simulink library "halout"  (R2021b)
settings: Solver=VariableStepAuto  StartTime=0.0  StopTime=10.0  RelTol=1e-3
undefined symbols (not defined in the file): C_TASK_5MS_S, FALSE, KHAL_CAN1FDAPS3E2E_flg, KHAL_CAN1FDAPS3TxReq_flg, KHAL_CAN1FDVCU2E2E_flg, KHAL_CAN1FDVCU2TxReq_flg, KHAL_CAN1FDVCU3E2E_flg, KHAL_CAN1FDVCU3TxReq_flg, KHAL_CAN1TxReq_flg, KHAL_CAN2TxReq_flg, KHAL_CAN3FDVCU1TxReq_flg, KHAL_CAN3FDVCU2E2E_flg, KHAL_CAN3FDVCU2TxReq_flg, KHAL_CAN3TxReq_flg, KHAL_CAN4FDVCU1E2E_flg, KHAL_CAN4FDVCU1TxReq_flg, KHAL_CAN4TxReq_flg, KHAL_CAN5TxReq_flg, ONE_INT, TRUE, ZERO_INT
libraries: FVT_lib x383, simulink x179
(part 20 of 20)

== system halout/HAL_OUT/CAN5/FD_VCU0_0x1F0/PwrStaSelect ==
  PwrStaSelect : Inport
  Data Type Conversion : DataTypeConversion  OutDataTypeStr=uint8  RndMeth=Round
  CAN5_PwrStaSelect : Outport
  wires:
  Data Type Conversion/1 -> CAN5_PwrStaSelect/1
  PwrStaSelect/1 -> Data Type Conversion/1

== system halout/HAL_OUT/CAN5/FD_VCU0_0x1F0/PwrStaTOSta ==
  PwrStaTOSta : Inport
  Data Type Conversion : DataTypeConversion  OutDataTypeStr=uint8  RndMeth=Round
  CAN5_PwrStaTOSta : Outport
  wires:
  Data Type Conversion/1 -> CAN5_PwrStaTOSta/1
  PwrStaTOSta/1 -> Data Type Conversion/1

== system halout/HAL_OUT/CAN5/FD_VCU0_0x1F0/PwrUpReq ==
  PwrUpReq : Inport
  Data Type Conversion : DataTypeConversion  OutDataTypeStr=uint8  RndMeth=Round
  CAN5_PwrUpReq : Outport
  wires:
  Data Type Conversion/1 -> CAN5_PwrUpReq/1
  PwrUpReq/1 -> Data Type Conversion/1

== system halout/HAL_OUT/CAN5/FD_VCU0_0x1F0/RrTqSource ==
  RrTqSource : Inport
  Data Type Conversion : DataTypeConversion  OutDataTypeStr=uint8  RndMeth=Round
  CAN5_Rr_TqSource : Outport
  wires:
  Data Type Conversion/1 -> CAN5_Rr_TqSource/1
  RrTqSource/1 -> Data Type Conversion/1

== system halout/HAL_OUT/CAN5/FD_VCU0_0x1F0/SchedChgTOSta ==
  SchedChgTOSta : Inport
  Data Type Conversion : DataTypeConversion  OutDataTypeStr=uint8  RndMeth=Round
  CAN5_SchedChgTOSta : Outport
  wires:
  Data Type Conversion/1 -> CAN5_SchedChgTOSta/1
  SchedChgTOSta/1 -> Data Type Conversion/1

== system halout/HAL_OUT/CAN5/FD_VCU0_0x1F0/SilentChkAllowSleep ==
  SilentChkAllowSleep : Inport
  Data Type Conversion : DataTypeConversion  OutDataTypeStr=uint8  RndMeth=Round
  CAN5_SilentChkAllowSleep : Outport
  wires:
  Data Type Conversion/1 -> CAN5_SilentChkAllowSleep/1
  SilentChkAllowSleep/1 -> Data Type Conversion/1

== system halout/HAL_OUT/CAN5/FD_VCU0_0x1F0/SysAllowReadySta ==
  SysAllowReadySta : Inport
  Data Type Conversion : DataTypeConversion  OutDataTypeStr=uint8  RndMeth=Round
  CAN5_SysAllowReadySta : Outport
  wires:
  Data Type Conversion/1 -> CAN5_SysAllowReadySta/1
  SysAllowReadySta/1 -> Data Type Conversion/1

== system halout/HAL_OUT/CAN5/FD_VCU0_0x1F0/SysPwrSta ==
  SysPwrSta : Inport
  Data Type Conversion : DataTypeConversion  OutDataTypeStr=uint8  RndMeth=Round
  CAN5_SysPwrSta : Outport
  wires:
  Data Type Conversion/1 -> CAN5_SysPwrSta/1
  SysPwrSta/1 -> Data Type Conversion/1

== system halout/HAL_OUT/CAN5/FD_VCU0_0x1F0/TCountSta ==
  TCountSta : Inport
  Data Type Conversion : DataTypeConversion  OutDataTypeStr=uint8  RndMeth=Round
  CAN5_TCountSta : Outport
  wires:
  Data Type Conversion/1 -> CAN5_TCountSta/1
  TCountSta/1 -> Data Type Conversion/1

== system halout/HAL_OUT/CAN5/FD_VCU0_0x1F0/TimerAllowSleep ==
  TimerAllowSleep : Inport
  Data Type Conversion : DataTypeConversion  OutDataTypeStr=uint8  RndMeth=Round
  CAN5_TimerAllowSleep : Outport
  wires:
  Data Type Conversion/1 -> CAN5_TimerAllowSleep/1
  TimerAllowSleep/1 -> Data Type Conversion/1

== system halout/HAL_OUT/CAN5/FD_VCU0_0x1F0/VCUBrkSWSta ==
  VCUBrkSWSta : Inport
  Data Type Conversion : DataTypeConversion  OutDataTypeStr=uint8  RndMeth=Round
  CAN5_VCUBrkSWSta : Outport
  wires:
  Data Type Conversion/1 -> CAN5_VCUBrkSWSta/1
  VCUBrkSWSta/1 -> Data Type Conversion/1

== system halout/HAL_OUT/CAN5/FD_VCU0_0x1F0/VCUFLDoorSta ==
  VCUFLDoorSta : Inport
  Data Type Conversion : DataTypeConversion  OutDataTypeStr=uint8  RndMeth=Round
  CAN5_VCUFLDoorSta : Outport
  wires:
  Data Type Conversion/1 -> CAN5_VCUFLDoorSta/1
  VCUFLDoorSta/1 -> Data Type Conversion/1

== system halout/HAL_OUT/CAN5/FD_VCU0_0x1F0/VCUFRDoorSta ==
  VCUFRDoorSta : Inport
  Data Type Conversion : DataTypeConversion  OutDataTypeStr=uint8  RndMeth=Round
  CAN5_VCUFRDoorSta : Outport
  wires:
  Data Type Conversion/1 -> CAN5_VCUFRDoorSta/1
  VCUFRDoorSta/1 -> Data Type Conversion/1

== system halout/HAL_OUT/CAN5/FD_VCU0_0x1F0/VCURLDoorSta ==
  VCURLDoorSta : Inport
  Data Type Conversion : DataTypeConversion  OutDataTypeStr=uint8  RndMeth=Round
  CAN5_VCURLDoorSta : Outport
  wires:
  Data Type Conversion/1 -> CAN5_VCURLDoorSta/1
  VCURLDoorSta/1 -> Data Type Conversion/1

== system halout/HAL_OUT/CAN5/FD_VCU0_0x1F0/VCURRDoorSta ==
  VCURRDoorSta : Inport
  Data Type Conversion : DataTypeConversion  OutDataTypeStr=uint8  RndMeth=Round
  CAN5_VCURRDoorSta : Outport
  wires:
  Data Type Conversion/1 -> CAN5_VCURRDoorSta/1
  VCURRDoorSta/1 -> Data Type Conversion/1

== system halout/HAL_OUT/CAN5/FD_VCU0_0x1F0/VehHVPwrAvail4THCM ==
  VehHVPwrAvail4THCM : Inport
  Data Type Conversion : DataTypeConversion  OutDataTypeStr=uint8  RndMeth=Round
  convert_out : FVT_lib/hal/convert_out  gain=50  offset=0
  CAN5_VehHVPwrAvail4THCM : Outport
  wires:
  Data Type Conversion/1 -> CAN5_VehHVPwrAvail4THCM/1
  convert_out/1 -> Data Type Conversion/1
  VehHVPwrAvail4THCM/1 -> convert_out/1

== system halout/HAL_OUT/CAN5/FD_VCU1_0x116/MSACrlSta ==
  MSACrlSta : Inport
  Data Type Conversion : DataTypeConversion  OutDataTypeStr=uint8  RndMeth=Round
  CAN5_MSA_Crl_Sta : Outport
  wires:
  Data Type Conversion/1 -> CAN5_MSA_Crl_Sta/1
  MSACrlSta/1 -> Data Type Conversion/1

== system halout/HAL_OUT/CAN5/FD_VCU1_0x116/PwrSta ==
  PwrSta : Inport
  Data Type Conversion : DataTypeConversion  OutDataTypeStr=uint8  RndMeth=Round
  CAN5_PwrSta : Outport
  wires:
  Data Type Conversion/1 -> CAN5_PwrSta/1
  PwrSta/1 -> Data Type Conversion/1

== system halout/HAL_OUT/CAN5/FD_VCU1_0x116/ShiftGearPosn ==
  ShiftGearPosn : Inport
  Data Type Conversion : DataTypeConversion  OutDataTypeStr=uint8  RndMeth=Round
  CAN5_ShiftGearPosn : Outport
  wires:
  Data Type Conversion/1 -> CAN5_ShiftGearPosn/1
  ShiftGearPosn/1 -> Data Type Conversion/1

== system halout/HAL_OUT/CAN5/FD_VCU3_0x159/CSVCU3CAN1 ==
  CSVCU3CAN1 : Inport
  Data Type Conversion : DataTypeConversion  OutDataTypeStr=uint8  RndMeth=Round
  CAN5_CS_VCU3_CAN1 : Outport
  wires:
  Data Type Conversion/1 -> CAN5_CS_VCU3_CAN1/1
  CSVCU3CAN1/1 -> Data Type Conversion/1

== system halout/HAL_OUT/CAN5/FD_VCU3_0x159/EquivAccPedalSWSta ==
  EquivAccPedalSWSta : Inport
  Data Type Conversion : DataTypeConversion  OutDataTypeStr=uint8  RndMeth=Round
  CAN5_EquivAccPedalSWSta : Outport
  wires:
  Data Type Conversion/1 -> CAN5_EquivAccPedalSWSta/1
  EquivAccPedalSWSta/1 -> Data Type Conversion/1

== system halout/HAL_OUT/CAN5/FD_VCU3_0x159/FrEDUActTqValid ==
  FrEDUActTqValid : Inport
  Data Type Conversion : DataTypeConversion  OutDataTypeStr=uint8  RndMeth=Round
  CAN5_Fr_EDUActTqValid : Outport
  wires:
  Data Type Conversion/1 -> CAN5_Fr_EDUActTqValid/1
  FrEDUActTqValid/1 -> Data Type Conversion/1

== system halout/HAL_OUT/CAN5/FD_VCU3_0x159/FrEDUAvailBrkRgnTq ==
  FrEDUAvailBrkRgnTq : Inport
  Data Type Conversion : DataTypeConversion  OutDataTypeStr=uint16  RndMeth=Round
  convert_out : FVT_lib/hal/convert_out  gain=0.5  offset=-5300
  CAN5_Fr_EDUAvailBrkRgnTq : Outport
  wires:
  Data Type Conversion/1 -> CAN5_Fr_EDUAvailBrkRgnTq/1
  convert_out/1 -> Data Type Conversion/1
  FrEDUAvailBrkRgnTq/1 -> convert_out/1

== system halout/HAL_OUT/CAN5/FD_VCU3_0x159/FrEDUAvailBrkRgnTqValid ==
  FrEDUAvailBrkRgnTqValid : Inport
  Data Type Conversion : DataTypeConversion  OutDataTypeStr=uint8  RndMeth=Round
  CAN5_Fr_EDUAvailBrkRgnTqValid : Outport
  wires:
  Data Type Conversion/1 -> CAN5_Fr_EDUAvailBrkRgnTqValid/1
  FrEDUAvailBrkRgnTqValid/1 -> Data Type Conversion/1

== system halout/HAL_OUT/CAN5/FD_VCU3_0x159/FrEDURealARgnTq ==
  FrEDURealARgnTq : Inport
  Data Type Conversion : DataTypeConversion  OutDataTypeStr=uint16  RndMeth=Round
  convert_out : FVT_lib/hal/convert_out  gain=1  offset=-5300
  CAN5_Fr_EDURealARgnTq : Outport
  wires:
  Data Type Conversion/1 -> CAN5_Fr_EDURealARgnTq/1
  convert_out/1 -> Data Type Conversion/1
  FrEDURealARgnTq/1 -> convert_out/1

== system halout/HAL_OUT/CAN5/FD_VCU3_0x159/FrEDURealDrvOrBRgnTq ==
  FrEDURealDrvOrBRgnTq : Inport
  Data Type Conversion : DataTypeConversion  OutDataTypeStr=uint16  RndMeth=Round
  convert_out : FVT_lib/hal/convert_out  gain=0.5  offset=-5300
  CAN5_Fr_EDURealDrvOrBRgnTq : Outport
  wires:
  Data Type Conversion/1 -> CAN5_Fr_EDURealDrvOrBRgnTq/1
  convert_out/1 -> Data Type Conversion/1
  FrEDURealDrvOrBRgnTq/1 -> convert_out/1

== system halout/HAL_OUT/CAN5/FD_VCU3_0x159/FrEDURolRgnTqValid ==
  FrEDURolRgnTqValid : Inport
  Data Type Conversion : DataTypeConversion  OutDataTypeStr=uint8  RndMeth=Round
  CAN5_Fr_EDURolRgnTqValid : Outport
  wires:
  Data Type Conversion/1 -> CAN5_Fr_EDURolRgnTqValid/1
  FrEDURolRgnTqValid/1 -> Data Type Conversion/1

== system halout/HAL_OUT/CAN5/FD_VCU3_0x159/FrEDUSpd ==
  FrEDUSpd : Inport
  Data Type Conversion : DataTypeConversion  OutDataTypeStr=uint16  RndMeth=Round
  convert_out : FVT_lib/hal/convert_out  gain=1  offset=-2000
  CAN5_Fr_EDUSpd : Outport
  wires:
  Data Type Conversion/1 -> CAN5_Fr_EDUSpd/1
  convert_out/1 -> Data Type Conversion/1
  FrEDUSpd/1 -> convert_out/1

== system halout/HAL_OUT/CAN5/FD_VCU3_0x159/FrEDUSpdValid ==
  FrEDUSpdValid : Inport
  Data Type Conversion : DataTypeConversion  OutDataTypeStr=uint8  RndMeth=Round
  CAN5_Fr_EDUSpdValid : Outport
  wires:
  Data Type Conversion/1 -> CAN5_Fr_EDUSpdValid/1
  FrEDUSpdValid/1 -> Data Type Conversion/1

== system halout/HAL_OUT/CAN5/FD_VCU3_0x159/FrRgnDecrSta ==
  FrRgnDecrSta : Inport
  Data Type Conversion : DataTypeConversion  OutDataTypeStr=uint8  RndMeth=Round
  CAN5_Fr_RgnDecrSta : Outport
  wires:
  Data Type Conversion/1 -> CAN5_Fr_RgnDecrSta/1
  FrRgnDecrSta/1 -> Data Type Conversion/1

== system halout/HAL_OUT/CAN5/FD_VCU3_0x159/FrRgnPermSta ==
  FrRgnPermSta : Inport
  Data Type Conversion : DataTypeConversion  OutDataTypeStr=uint8  RndMeth=Round
  CAN5_Fr_RgnPermSta : Outport
  wires:
  Data Type Conversion/1 -> CAN5_Fr_RgnPermSta/1
  FrRgnPermSta/1 -> Data Type Conversion/1

== system halout/HAL_OUT/CAN5/FD_VCU3_0x159/PTCSPermSta ==
  PTCSPermSta : Inport
  Data Type Conversion : DataTypeConversion  OutDataTypeStr=uint8  RndMeth=Round
  CAN5_PTCS_PermSta : Outport
  wires:
  Data Type Conversion/1 -> CAN5_PTCS_PermSta/1
  PTCSPermSta/1 -> Data Type Conversion/1

== system halout/HAL_OUT/CAN5/FD_VCU3_0x159/RCVCU3CAN1 ==
  RCVCU3CAN1 : Inport
  Data Type Conversion : DataTypeConversion  OutDataTypeStr=uint8  RndMeth=Round
  CAN5_RC_VCU3_CAN1 : Outport
  wires:
  Data Type Conversion/1 -> CAN5_RC_VCU3_CAN1/1
  RCVCU3CAN1/1 -> Data Type Conversion/1

== system halout/HAL_OUT/CAN5/FD_VCU3_0x159/RgnAbnorSta ==
  RgnAbnorSta : Inport
  Data Type Conversion : DataTypeConversion  OutDataTypeStr=uint8  RndMeth=Round
  CAN5_RgnAbnorSta : Outport
  wires:
  Data Type Conversion/1 -> CAN5_RgnAbnorSta/1
  RgnAbnorSta/1 -> Data Type Conversion/1

== system halout/HAL_OUT/CAN5/FD_VCU3_0x159/RrEDUActTqValid ==
  RrEDUActTqValid : Inport
  Data Type Conversion : DataTypeConversion  OutDataTypeStr=uint8  RndMeth=Round
  CAN5_Rr_EDUActTqValid : Outport
  wires:
  Data Type Conversion/1 -> CAN5_Rr_EDUActTqValid/1
  RrEDUActTqValid/1 -> Data Type Conversion/1

== system halout/HAL_OUT/CAN5/FD_VCU3_0x159/RrEDUAvailBrkRgnTq ==
  RrEDUAvailBrkRgnTq : Inport
  Data Type Conversion : DataTypeConversion  OutDataTypeStr=uint16  RndMeth=Round
  convert_out : FVT_lib/hal/convert_out  gain=0.5  offset=-5300
  CAN5_Rr_EDUAvailBrkRgnTq : Outport
  wires:
  Data Type Conversion/1 -> CAN5_Rr_EDUAvailBrkRgnTq/1
  convert_out/1 -> Data Type Conversion/1
  RrEDUAvailBrkRgnTq/1 -> convert_out/1

== system halout/HAL_OUT/CAN5/FD_VCU3_0x159/RrEDUAvailBrkRgnTqValid ==
  RrEDUAvailBrkRgnTqValid : Inport
  Data Type Conversion : DataTypeConversion  OutDataTypeStr=uint8  RndMeth=Round
  CAN5_Rr_EDUAvailBrkRgnTqValid : Outport
  wires:
  Data Type Conversion/1 -> CAN5_Rr_EDUAvailBrkRgnTqValid/1
  RrEDUAvailBrkRgnTqValid/1 -> Data Type Conversion/1

== system halout/HAL_OUT/CAN5/FD_VCU3_0x159/RrEDURealARgnTq ==
  RrEDURealARgnTq : Inport
  Data Type Conversion : DataTypeConversion  OutDataTypeStr=uint16  RndMeth=Round
  convert_out : FVT_lib/hal/convert_out  gain=1  offset=-5300
  CAN5_Rr_EDURealARgnTq : Outport
  wires:
  Data Type Conversion/1 -> CAN5_Rr_EDURealARgnTq/1
  convert_out/1 -> Data Type Conversion/1
  RrEDURealARgnTq/1 -> convert_out/1

== system halout/HAL_OUT/CAN5/FD_VCU3_0x159/RrEDURealDrvOrBRgnTq ==
  RrEDURealDrvOrBRgnTq : Inport
  Data Type Conversion : DataTypeConversion  OutDataTypeStr=uint16  RndMeth=Round
  convert_out : FVT_lib/hal/convert_out  gain=0.5  offset=-5300
  CAN5_Rr_EDURealDrvOrBRgnTq : Outport
  wires:
  Data Type Conversion/1 -> CAN5_Rr_EDURealDrvOrBRgnTq/1
  convert_out/1 -> Data Type Conversion/1
  RrEDURealDrvOrBRgnTq/1 -> convert_out/1

== system halout/HAL_OUT/CAN5/FD_VCU3_0x159/RrEDURolRgnTqValid ==
  RrEDURolRgnTqValid : Inport
  Data Type Conversion : DataTypeConversion  OutDataTypeStr=uint8  RndMeth=Round
  CAN5_Rr_EDURolRgnTqValid : Outport
  wires:
  Data Type Conversion/1 -> CAN5_Rr_EDURolRgnTqValid/1
  RrEDURolRgnTqValid/1 -> Data Type Conversion/1

== system halout/HAL_OUT/CAN5/FD_VCU3_0x159/RrEDUSpd ==
  RrEDUSpd : Inport
  Data Type Conversion : DataTypeConversion  OutDataTypeStr=uint16  RndMeth=Round
  convert_out : FVT_lib/hal/convert_out  gain=1  offset=-2000
  CAN5_Rr_EDUSpd : Outport
  wires:
  Data Type Conversion/1 -> CAN5_Rr_EDUSpd/1
  convert_out/1 -> Data Type Conversion/1
  RrEDUSpd/1 -> convert_out/1

== system halout/HAL_OUT/CAN5/FD_VCU3_0x159/RrEDUSpdValid ==
  RrEDUSpdValid : Inport
  Data Type Conversion : DataTypeConversion  OutDataTypeStr=uint8  RndMeth=Round
  CAN5_Rr_EDUSpdValid : Outport
  wires:
  Data Type Conversion/1 -> CAN5_Rr_EDUSpdValid/1
  RrEDUSpdValid/1 -> Data Type Conversion/1

== system halout/HAL_OUT/CAN5/FD_VCU3_0x159/RrRgnDecrSta ==
  RrRgnDecrSta : Inport
  Data Type Conversion : DataTypeConversion  OutDataTypeStr=uint8  RndMeth=Round
  CAN5_Rr_RgnDecrSta : Outport
  wires:
  Data Type Conversion/1 -> CAN5_Rr_RgnDecrSta/1
  RrRgnDecrSta/1 -> Data Type Conversion/1

== system halout/HAL_OUT/CAN5/FD_VCU3_0x159/RrRgnPermSta ==
  RrRgnPermSta : Inport
  Data Type Conversion : DataTypeConversion  OutDataTypeStr=uint8  RndMeth=Round
  CAN5_Rr_RgnPermSta : Outport
  wires:
  Data Type Conversion/1 -> CAN5_Rr_RgnPermSta/1
  RrRgnPermSta/1 -> Data Type Conversion/1

== system halout/HAL_OUT/CAN5/FD_VCU4_0x3C0/EngAGSCloseSta ==
  EngAGSCloseSta : Inport
  Data Type Conversion : DataTypeConversion  OutDataTypeStr=uint8  RndMeth=Round
  CAN5_Eng_AGSCloseSta : Outport
  wires:
  Data Type Conversion/1 -> CAN5_Eng_AGSCloseSta/1
  EngAGSCloseSta/1 -> Data Type Conversion/1

== system halout/HAL_OUT/CAN5/FD_VCU4_0x3C0/EngActvDmpDisabSta ==
  EngActvDmpDisabSta : Inport
  Data Type Conversion : DataTypeConversion  OutDataTypeStr=uint8  RndMeth=Round
  CAN5_Eng_ActvDmpDisabSta : Outport
  wires:
  Data Type Conversion/1 -> CAN5_Eng_ActvDmpDisabSta/1
  EngActvDmpDisabSta/1 -> Data Type Conversion/1

== system halout/HAL_OUT/CAN5/FD_VCU4_0x3C0/EngCoastDwSta ==
  EngCoastDwSta : Inport
  Data Type Conversion : DataTypeConversion  OutDataTypeStr=uint8  RndMeth=Round
  CAN5_Eng_CoastDwSta : Outport
  wires:
  Data Type Conversion/1 -> CAN5_Eng_CoastDwSta/1
  EngCoastDwSta/1 -> Data Type Conversion/1

== system halout/HAL_OUT/CAN5/FD_VCU4_0x3C0/EngPwrLockSta ==
  EngPwrLockSta : Inport
  Data Type Conversion : DataTypeConversion  OutDataTypeStr=uint8  RndMeth=Round
  CAN5_Eng_PwrLockSta : Outport
  wires:
  Data Type Conversion/1 -> CAN5_Eng_PwrLockSta/1
  EngPwrLockSta/1 -> Data Type Conversion/1

== system halout/HAL_OUT/CAN5/FD_VCU4_0x3C0/VehMalfunLevel ==
  VehMalfunLevel : Inport
  Data Type Conversion : DataTypeConversion  OutDataTypeStr=uint8  RndMeth=Round
  CAN5_VehMalfunLevel : Outport
  wires:
  Data Type Conversion/1 -> CAN5_VehMalfunLevel/1
  VehMalfunLevel/1 -> Data Type Conversion/1

== system halout/HAL_OUT/CAN5/FD_VCU5_0x245/EDriveSysErrAccPedalErr ==
  EDriveSysErrAccPedalErr : Inport
  Data Type Conversion : DataTypeConversion  OutDataTypeStr=uint8  RndMeth=Round
  CAN5_EDriveSysErr_AccPedalErr : Outport
  wires:
  Data Type Conversion/1 -> CAN5_EDriveSysErr_AccPedalErr/1
  EDriveSysErrAccPedalErr/1 -> Data Type Conversion/1

== system halout/HAL_OUT/CAN5/FD_VCU5_0x245/EDriveSysErrMCUErr ==
  EDriveSysErrMCUErr : Inport
  Data Type Conversion : DataTypeConversion  OutDataTypeStr=uint8  RndMeth=Round
  CAN5_EDriveSysErr_MCUErr : Outport
  wires:
  Data Type Conversion/1 -> CAN5_EDriveSysErr_MCUErr/1
  EDriveSysErrMCUErr/1 -> Data Type Conversion/1

== system halout/HAL_OUT/CAN5/FD_VCU5_0x245/EDriveSysErrShifterErr ==
  EDriveSysErrShifterErr : Inport
  Data Type Conversion : DataTypeConversion  OutDataTypeStr=uint8  RndMeth=Round
  CAN5_EDriveSysErr_ShifterErr : Outport
  wires:
  Data Type Conversion/1 -> CAN5_EDriveSysErr_ShifterErr/1
  EDriveSysErrShifterErr/1 -> Data Type Conversion/1

== system halout/HAL_OUT/CAN5/FD_VCU5_0x245/EDriveSysErrVCUErr ==
  EDriveSysErrVCUErr : Inport
  Data Type Conversion : DataTypeConversion  OutDataTypeStr=uint8  RndMeth=Round
  CAN5_EDriveSysErr_VCUErr : Outport
  wires:
  Data Type Conversion/1 -> CAN5_EDriveSysErr_VCUErr/1
  EDriveSysErrVCUErr/1 -> Data Type Conversion/1

== system halout/HAL_OUT/CAN5/FD_VCU5_0x245/HVSysErrIsolationErr ==
  HVSysErrIsolationErr : Inport
  Data Type Conversion : DataTypeConversion  OutDataTypeStr=uint8  RndMeth=Round
  CAN5_HVSysErr_IsolationErr : Outport
  wires:
  Data Type Conversion/1 -> CAN5_HVSysErr_IsolationErr/1
  HVSysErrIsolationErr/1 -> Data Type Conversion/1

== system halout/HAL_OUT/CAN5/FD_VCU5_0x245/HVSysErrPackErr ==
  HVSysErrPackErr : Inport
  Data Type Conversion : DataTypeConversion  OutDataTypeStr=uint8  RndMeth=Round
  CAN5_HVSysErr_PackErr : Outport
  wires:
  Data Type Conversion/1 -> CAN5_HVSysErr_PackErr/1
  HVSysErrPackErr/1 -> Data Type Conversion/1

== system halout/HAL_OUT/CAN5/FD_VCU5_0x245/HVSysErrRelayErr ==
  HVSysErrRelayErr : Inport
  Data Type Conversion : DataTypeConversion  OutDataTypeStr=uint8  RndMeth=Round
  CAN5_HVSysErr_RelayErr : Outport
  wires:
  Data Type Conversion/1 -> CAN5_HVSysErr_RelayErr/1
  HVSysErrRelayErr/1 -> Data Type Conversion/1

== system halout/HAL_OUT/CAN5/FD_VCU5_0x245/LVSysErrPwrOutpErr ==
  LVSysErrPwrOutpErr : Inport
  Data Type Conversion : DataTypeConversion  OutDataTypeStr=uint8  RndMeth=Round
  CAN5_LVSysErr_PwrOutpErr : Outport
  wires:
  Data Type Conversion/1 -> CAN5_LVSysErr_PwrOutpErr/1
  LVSysErrPwrOutpErr/1 -> Data Type Conversion/1

== system halout/HAL_OUT/CAN5/FD_VCU5_0x245/LimphomeAct ==
  LimphomeAct : Inport
  Data Type Conversion : DataTypeConversion  OutDataTypeStr=uint8  RndMeth=Round
  CAN5_LimphomeAct : Outport
  wires:
  Data Type Conversion/1 -> CAN5_LimphomeAct/1
  LimphomeAct/1 -> Data Type Conversion/1

== system halout/HAL_OUT/CAN5/FD_VCU5_0x245/LowSOCWarn ==
  LowSOCWarn : Inport
  Data Type Conversion : DataTypeConversion  OutDataTypeStr=uint8  RndMeth=Round
  CAN5_LowSOCWarn : Outport
  wires:
  Data Type Conversion/1 -> CAN5_LowSOCWarn/1
  LowSOCWarn/1 -> Data Type Conversion/1

== system halout/HAL_OUT/CAN5/FD_VCU5_0x245/PwrStaErr ==
  PwrStaErr : Inport
  Data Type Conversion : DataTypeConversion  OutDataTypeStr=uint8  RndMeth=Round
  CAN5_PwrStaErr : Outport
  wires:
  Data Type Conversion/1 -> CAN5_PwrStaErr/1
  PwrStaErr/1 -> Data Type Conversion/1

== system halout/HAL_OUT/CAN5/FD_VCU5_0x245/ReVehThdChkSta ==
  ReVehThdChkSta : Inport
  Data Type Conversion : DataTypeConversion  OutDataTypeStr=uint8  RndMeth=Round
  CAN5_Re_VehThdChkSta : Outport
  wires:
  Data Type Conversion/1 -> CAN5_Re_VehThdChkSta/1
  ReVehThdChkSta/1 -> Data Type Conversion/1

== stateflow chart halout/HAL_OUT/CAN1/FD_VCU2_Tx/Chart ==
  state TrigCounter
    en:
    counter = 0;
    counter++;
    (default) -> (junction 5)
    TrigCounter -> (junction 5) : {
        | counter++;
        | }
    (junction 5) -> (junction 6) [order 1] : [TxReq && (counter %% CycleCnt) == 0]
    (junction 5) -> (junction 7) [order 2]
    (junction 6) -> (junction 8) : {
        | TxTrigger;
        | counter = 0;
        | }
    (junction 8) -> (junction 7)
    (junction 7) -> (junction 34)
    (junction 34) -> (junction 33) [order 1] : [ !TxReq]
    (junction 34) -> (junction 35) [order 2]
    (junction 33) -> (junction 36) : {
        | counter = 0;
        | }
    (junction 36) -> (junction 35)
    (junction 35) -> (junction 44)
  data: TxReq input; CycleCnt input; counter local uint16
  events: TxTrigger output FUNCTION_CALL_EVENT

== stateflow chart halout/HAL_OUT/CAN1/FD_VCU3_Tx/Chart ==
  state TrigCounter
    en:
    counter = 0;
    counter++;
    (default) -> (junction 5)
    TrigCounter -> (junction 5) : {
        | counter++;
        | }
    (junction 5) -> (junction 6) [order 1] : [TxReq && (counter %% CycleCnt) == 0]
    (junction 5) -> (junction 7) [order 2]
    (junction 6) -> (junction 8) : {
        | TxTrigger;
        | counter = 0;
        | }
    (junction 8) -> (junction 7)
    (junction 7) -> (junction 34)
    (junction 34) -> (junction 33) [order 1] : [ !TxReq]
    (junction 34) -> (junction 35) [order 2]
    (junction 33) -> (junction 36) : {
        | counter = 0;
        | }
    (junction 36) -> (junction 35)
    (junction 35) -> (junction 44)
  data: TxReq input; CycleCnt input; counter local uint16
  events: TxTrigger output FUNCTION_CALL_EVENT

== stateflow chart halout/HAL_OUT/CAN1/FD_APS3_Tx/Chart ==
  state TrigCounter
    en:
    counter = 0;
    counter++;
    (default) -> (junction 5)
    TrigCounter -> (junction 5) : {
        | counter++;
        | }
    (junction 5) -> (junction 6) [order 1] : [TxReq && (counter %% CycleCnt) == 0]
    (junction 5) -> (junction 7) [order 2]
    (junction 6) -> (junction 8) : {
        | TxTrigger;
        | counter = 0;
        | }
    (junction 8) -> (junction 7)
    (junction 7) -> (junction 34)
    (junction 34) -> (junction 33) [order 1] : [ !TxReq]
    (junction 34) -> (junction 35) [order 2]
    (junction 33) -> (junction 36) : {
        | counter = 0;
        | }
    (junction 36) -> (junction 35)
    (junction 35) -> (junction 44)
  data: TxReq input; CycleCnt input; counter local uint16
  events: TxTrigger output FUNCTION_CALL_EVENT

== stateflow chart halout/HAL_OUT/CAN3/FD_VCU1_Tx/Chart1 ==
  state TrigCounter
    en:
    counter = 0;
    counter++;
    (default) -> (junction 5)
    TrigCounter -> (junction 5) : {
        | counter++;
        | TxTrigger = FALSE;
        | CycleTriggerred = FALSE;
        | }
    (junction 5) -> (junction 6) [order 1] : [TxReq && (counter %% CycleCnt) == 0]
    (junction 5) -> (junction 7) [order 2]
    (junction 6) -> (junction 8) : {
        | TxTrigger = TRUE;
        | counter = 0;
        | CycleTriggerred =TRUE;
        | }
    (junction 8) -> (junction 7)
    (junction 7) -> (junction 34)
    (junction 34) -> (junction 38) [order 1] : [TxReq && EventReq && !CycleTriggerred]
    (junction 34) -> (junction 36) [order 2]
    (junction 38) -> (junction 40) : {
        | TxTrigger = TRUE;
        | }
    (junction 40) -> (junction 36)
    (junction 36) -> (junction 21)
    (junction 21) -> (junction 23) [order 1] : [ !TxReq]
    (junction 21) -> (junction 22) [order 2]
    (junction 23) -> (junction 20) : {
        | counter = 0;
        | }
    (junction 20) -> (junction 22)
    (junction 22) -> (junction 31)
  data: TxReq input; EventReq input; CycleCnt input; counter local uint16; CycleTriggerred local boolean; FALSE parameter; TRUE parameter; TxTrigger output double

== stateflow chart halout/HAL_OUT/CAN3/FD_VCU2_Tx/Chart ==
  state TrigCounter
    en:
    counter = 0;
    counter++;
    (default) -> (junction 5)
    TrigCounter -> (junction 5) : {
        | counter++;
        | }
    (junction 5) -> (junction 6) [order 1] : [TxReq && (counter %% CycleCnt) == 0]
    (junction 5) -> (junction 7) [order 2]
    (junction 6) -> (junction 8) : {
        | TxTrigger;
        | counter = 0;
        | }
    (junction 8) -> (junction 7)
    (junction 7) -> (junction 34)
    (junction 34) -> (junction 33) [order 1] : [ !TxReq]
    (junction 34) -> (junction 35) [order 2]
    (junction 33) -> (junction 36) : {
        | counter = 0;
        | }
    (junction 36) -> (junction 35)
    (junction 35) -> (junction 44)
  data: TxReq input; CycleCnt input; counter local uint16
  events: TxTrigger output FUNCTION_CALL_EVENT

== stateflow chart halout/HAL_OUT/CAN4/FD_VCU1_Tx/Chart ==
  state TrigCounter
    en:
    counter = 0;
    counter++;
    (default) -> (junction 55) : {DelayWorkaround = 0;}
    TrigCounter -> (junction 55) : {
        | counter++;
        | CycleTriggerred = FALSE;
        | DelayWorkaround++;
        | }
    (junction 55) -> (junction 31) [order 2]
    (junction 55) -> (junction 5) [order 1] : [DelayWorkaround >= 0]{DelayWorkaround = 0;}
    (junction 5) -> (junction 6) [order 1] : [TxReq && (counter %% CycleCnt) == 0]
    (junction 5) -> (junction 7) [order 2]
    (junction 6) -> (junction 8) : {
        | TriggerDataUpdate;
        | TriggerCallCDD;
        | counter = 0;
        | CycleTriggerred =TRUE;
        | }
    (junction 8) -> (junction 7)
    (junction 7) -> (junction 34)
    (junction 34) -> (junction 38) [order 1] : [TxReq && EventReq && !CycleTriggerred]
    (junction 34) -> (junction 36) [order 2]
    (junction 38) -> (junction 40) : {
        | TriggerDataUpdate;
        | TriggerCallCDD;
        | }
    (junction 40) -> (junction 36)
    (junction 36) -> (junction 21)
    (junction 21) -> (junction 23) [order 1] : [ !TxReq]
    (junction 21) -> (junction 22) [order 2]
    (junction 23) -> (junction 20) : {
        | counter = 0;
        | }
    (junction 20) -> (junction 22)
    (junction 22) -> (junction 31)
  data: TxReq input; EventReq input; CycleCnt input; counter local uint16; CycleTriggerred local boolean; FALSE parameter; TRUE parameter; DelayWorkaround local double
  events: TriggerDataUpdate output FUNCTION_CALL_EVENT; TriggerCallCDD output FUNCTION_CALL_EVENT

== stateflow chart halout/HAL_OUT/CAN_Scheduler ==
  state CAN_scheduler
    (default) -> (junction 55)
    CAN_scheduler -> (junction 55)
    (junction 55) -> (junction 53) [order 1] : [KHAL_CAN1TxReq_flg && VOUTP_ALLCANTxReq_flg]
    (junction 55) -> (junction 214) [order 2]
    (junction 53) -> (junction 212) : {
        | trig_can1;
        | }
    (junction 212) -> (junction 214)
    (junction 214) -> (junction 250)
    (junction 250) -> (junction 251) [order 1] : [KHAL_CAN2TxReq_flg && VOUTP_ALLCANTxReq_flg]
    (junction 250) -> (junction 253) [order 2]
    (junction 251) -> (junction 247) : {
        | trig_can2;
        | }
    (junction 247) -> (junction 253)
    (junction 253) -> (junction 258)
    (junction 258) -> (junction 259) [order 1] : [KHAL_CAN3TxReq_flg && VOUTP_ALLCANTxReq_flg]
    (junction 258) -> (junction 261) [order 2]
    (junction 259) -> (junction 255) : {
        | trig_can3;
        | }
    (junction 255) -> (junction 261)
    (junction 261) -> (junction 266)
    (junction 266) -> (junction 267) [order 1] : [KHAL_CAN4TxReq_flg && VOUTP_ALLCANTxReq_flg]
    (junction 266) -> (junction 269) [order 2]
    (junction 267) -> (junction 263) : {
        | trig_can4;
        | }
    (junction 263) -> (junction 269)
    (junction 269) -> (junction 274)
    (junction 274) -> (junction 275) [order 1] : [KHAL_CAN5TxReq_flg && VOUTP_ALLCANTxReq_flg]
    (junction 274) -> (junction 277) [order 2]
    (junction 275) -> (junction 271) : {
        | trig_can5;
        | }
    (junction 271) -> (junction 277)
  data: KHAL_CAN1TxReq_flg input; KHAL_CAN2TxReq_flg input; KHAL_CAN3TxReq_flg input; KHAL_CAN4TxReq_flg input; KHAL_CAN5TxReq_flg input; VOUTP_ALLCANTxReq_flg input
  events: trig_can1 output FUNCTION_CALL_EVENT; trig_can2 output FUNCTION_CALL_EVENT; trig_can3 output FUNCTION_CALL_EVENT; trig_can4 output FUNCTION_CALL_EVENT; trig_can5 output FUNCTION_CALL_EVENT
